simulink model "DriveTrain_SystemID"  (R2019a)
settings: Solver=VariableStepAuto  StartTime=0.0  StopTime=90.0  MaxStep=Ts*10  RelTol=1e-3
InitFcn:
  | %DriveTrainInitialise;
values from neighbouring files (symbols this model uses):
  PolePairs = 10    [DrivetrainParametersForRhys.m]
undefined symbols (not defined in the file or in its folder): Iq_max, RotorInertia
libraries: nesl_utility x6, fl_lib x4, ee_lib x2, MotorLIB x2, powerlib_meascontrol x1, eeTransforms x1
settings Model: OrderedModelArguments=off  Creator=plewi  LastModifiedBy=plewi

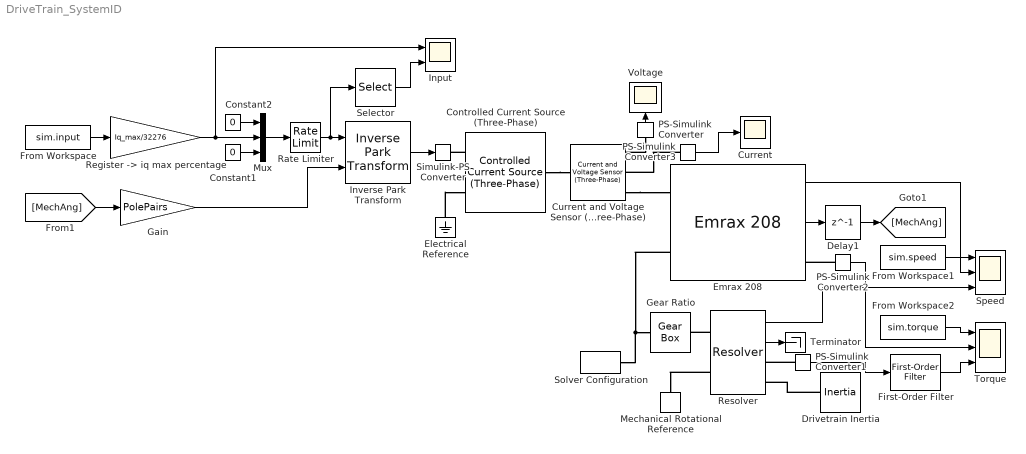
== system DriveTrain_SystemID ==
  Constant1 : Constant  Value=0
  Constant2 : Constant  Value=0
  Controlled Current Source (Three-Phase) : ee_lib/Sources/Controlled Current Source (Three-Phase)
      settings: SourceProductName=Simscape Electrical  SourceProductBaseCode=PS
  Current : Scope
  Current and Voltage Sensor (Three-Phase) : ee_lib/Sensors & Transducers/Current and Voltage Sensor (Three-Phase)  vMeasurementType=ee.enum.vmeasurement.lg  outputUnit=ee.enum.unit.si  SRated=100e6 V*A  VRated=24e3 V  I_specify=off  I_priority=None  I=[ 0 0 0 ] A  I_nominal_specify=off  I_nominal_unit=A  I_nominal_value=1  V_specify=off  V_priority=None  V=[ 0 0 0 ] V  V_nominal_specify=off  V_nominal_unit=V  V_nominal_value=1
      settings: SourceProductName=Simscape Electrical  SourceProductBaseCode=PS
  Delay1 : Delay  DelayLength=1
  Drivetrain Inertia : fl_lib/Mechanical/Rotational Elements/Inertia  inertia=J kg*m^2  w_specify=off  w_priority=High  w=0 rad/s  w_nominal_specify=off  w_nominal_unit=rad/s  w_nominal_value=1  t_specify=off  t_priority=None  t=0 N*m  t_nominal_specify=off  t_nominal_unit=N*m  t_nominal_value=1
  Electrical Reference : fl_lib/Electrical/Electrical Elements/Electrical Reference
  Emrax 208 : MotorLIB/Emrax 208  nPolePairs=PolePairs  pm_flux_linkage=PM  Ld=Ld  Lq=Lq  L0=2e-4  Rs=Rs  zero_sequence=ee.enum.park.zerosequence.exclude  J=RotorInertia
  First-Order Filter : powerlib_meascontrol/Filters/First-Order Filter  FilterType=Lowpass  Tc=1  Ts=0  Initialize=on  Vac_Init=[0, 0, 60]  Vdc_Init=0  PlotResponse=off  FreqRange="[0,  200,  1]"
      settings: SourceProductName=Simscape Electrical
  From Workspace : FromWorkspace  VariableName=sim.input  SampleTime=0
  From Workspace1 : FromWorkspace  VariableName=sim.speed  SampleTime=0
  From Workspace2 : FromWorkspace  VariableName=sim.torque  SampleTime=0
  Gain : Gain  Gain=PolePairs
  Gear Ratio : fl_lib/Mechanical/Mechanisms/Gear Box  ratio=3.27  t_in_specify=off  t_in_priority=None  t_in=0 N*m  t_in_nominal_specify=off  t_in_nominal_unit=N*m  t_in_nominal_value=1  t_out_specify=off  t_out_priority=None  t_out=0 N*m  t_out_nominal_specify=off  t_out_nominal_unit=N*m  t_out_nominal_value=1
  Input : Scope  NumInputPorts=2
  Inverse Park Transform : eeTransforms/Inverse Park Transform  AxisAlignment=Q-axis  PowerInvariant=off
      settings: SourceProductName=Simscape Electrical
  Mechanical Rotational Reference : fl_lib/Mechanical/Rotational Elements/Mechanical Rotational Reference
  Mux : Mux  Inputs=3
  PS-Simulink Converter{,1..3} (4 alike) : nesl_utility/PS-Simulink Converter  PhysicalDomain=network_engine_domain  SubClassName=ps_output  LeftPortType=input  RightPortType=output  PseudoPeriodic=off  Frequencies=[]  Unit=1  AffineConversion=off
  Rate Limiter : RateLimiter  RisingSlewLimit=10  FallingSlewLimit=-10  SampleTimeMode=inherited
  "Register -> iq max percentage" : Gain  Gain=Iq_max/32276
  Resolver : MotorLIB/Emrax 208/Resolver  SystemSampleTime=-1
  Selector : Selector  InputPortWidth=3  IndexOptions=Index vector (dialog)  Indices=[2]  OutputSizes=1
  Simulink-PS Converter : nesl_utility/Simulink-PS Converter  PhysicalDomain=network_engine_domain  SubClassName=ps_input  LeftPortType=input  RightPortType=output  PseudoPeriodic=off  Frequencies=[]  NoiseDistribution=none  NoiseParameters=[]  Unit=1  AffineConversion=off  FilteringAndDerivatives=provide  SimscapeFilterOrder=1  InputFilterTimeConstant=0.001  UdotUserProvided=0
  Solver Configuration : nesl_utility/Solver Configuration  PhysicalDomain=network_engine_domain  SubClassName=solver  LeftPortType=input  RightPortType=generic  Tones=[]  Harmonics=[]  SimulateNoise=off  Profile=off  UseLocalSampling=off  EnableSwitchedLinearOptims=on  FrequencyDomain=off  UseCCode=off  RelTol=0.001  AbsTol=1e-06  MinStep=1e-09  ToWorkspace=off  RevertToSquareIcSolve=off  NumHomotopyIterations=100  PhasorMode=off  PhasorModeNumHarmonics=1  DoDC=off  ResidualTolerance=1e-09  UseLocalSolver=off  LocalSolverChoice=NE_BACKWARD_EULER_ADVANCER  LocalSolverSampleTime=0.001  DoFixedCost=off  MaxNonlinIter=3  MaxModeIter=2  LinearAlgebra=auto  EquationFormulation=NE_TIME_EF  DelaysMemoryBudget=1024  AutomaticFiltering=on  FilteringTimeConstant=0.001  PartitionStorageMethod=AS_NEEDED  PartitionMemoryBudget=1024  PartitionMethod=ROBUST
  Speed : Scope  NumInputPorts=3
  Terminator : Terminator
  Torque : Scope  NumInputPorts=3
  Voltage : Scope
  wires:
  Inverse Park Transform/1 -> Simulink-PS Converter/1
  Resolver/2 -> Terminator/1
  [MechAng] -> Gain/1
  Gain/1 -> Inverse Park Transform/2
  Emrax 208/2 -> Delay1/1
  Delay1/1 -> [MechAng]
  PS-Simulink Converter2/1 -> Torque/2
  From Workspace/1 -> "Register -> iq max percentage"/1
  Constant1/1 -> Mux/3
  "Register -> iq max percentage"/1 -> Input/1, Mux/2
  Constant2/1 -> Mux/1
  PS-Simulink Converter/1 -> Voltage/1
  Resolver/1 -> Speed/3
  Emrax 208/1 -> Speed/2
  From Workspace1/1 -> Speed/1
  From Workspace2/1 -> Torque/1
  PS-Simulink Converter3/1 -> Current/1
  Mux/1 -> Rate Limiter/1
  Rate Limiter/1 -> Selector/1, Inverse Park Transform/1
  Selector/1 -> Input/2
  PS-Simulink Converter1/1 -> First-Order Filter/1
  First-Order Filter/1 -> Torque/3
  connections:
  Electrical Reference/LConn1 -- Controlled Current Source (Three-Phase)/LConn2
  Gear Ratio/LConn1 -- Emrax 208/LConn2 -- Solver Configuration/RConn1
  PS-Simulink Converter1/LConn1 -- Resolver/RConn1
  Drivetrain Inertia/LConn1 -- Resolver/RConn2
  Resolver/LConn2 -- Mechanical Rotational Reference/LConn1
  Resolver/LConn1 -- Gear Ratio/RConn1
  PS-Simulink Converter2/LConn1 -- Emrax 208/RConn1
  Current and Voltage Sensor (Three-Phase)/RConn3 -- Emrax 208/LConn1
  PS-Simulink Converter/LConn1 -- Current and Voltage Sensor (Three-Phase)/RConn1
  PS-Simulink Converter3/LConn1 -- Current and Voltage Sensor (Three-Phase)/RConn2
  Controlled Current Source (Three-Phase)/RConn1 -- Current and Voltage Sensor (Three-Phase)/LConn1
  Controlled Current Source (Three-Phase)/LConn1 -- Simulink-PS Converter/RConn1
